simulink model "Fcn1"  (R2017b)
settings: Solver=FixedStepDiscrete  StartTime=0.0  StopTime=10  FixedStep=0.200000  RelTol=1e-3  EnableMultiTasking=on
settings Model: Creator=ktrinh  LastModifiedBy=hbourbou
settings DataIOCC: SaveFormat=Structure
settings OptimizationCC: LifeSpan=inf
settings DebuggingCC: SFUnexpectedBacktrackingDiag=warning  SFNoUnconditionalDefaultTransitionDiag=warning  SFExecutionAtInitializationDiag=none
settings HardwareCC: ProdBitPerSizeT=32  ProdBitPerPtrDiffT=32  ProdWordSize=32  ProdHWDeviceType=Specified
settings CodeAppCC: StateflowObjectComments=on
settings GRTTargetCC: TargetLangStandard=C89/C90 (ANSI)  GeneratePreprocessorConditionals=Disable all
settings ConfigComp: CovMetricSettings=dw  CovHtmlReporting=on  CovSaveCumulativeToWorkspaceVar=on  CovSaveSingleToWorkspaceVar=on  CovExternalEMLEnable=off

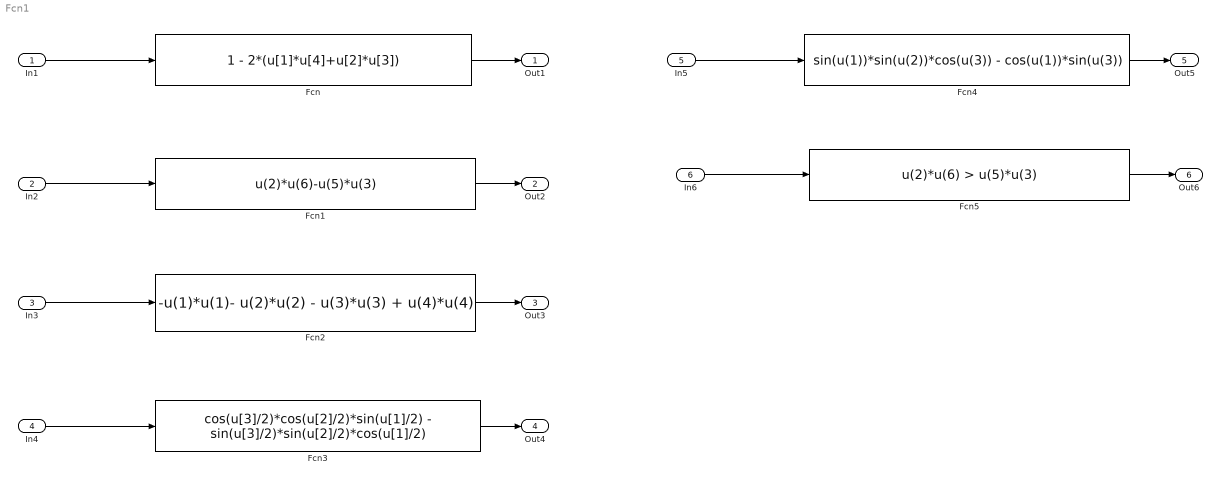
== system Fcn1 ==
  In1 : Inport  PortDimensions=4
  In2 : Inport  Port=2  PortDimensions=6
  In3 : Inport  Port=3  PortDimensions=4
  In4 : Inport  Port=4  PortDimensions=3
  In5 : Inport  Port=5  PortDimensions=3
  In6 : Inport  Port=6  PortDimensions=6
  Fcn : Fcn  Expr=1 - 2*(u[1]*u[4]+u[2]*u[3])
  Fcn1 : Fcn  Expr=u(2)*u(6)-u(5)*u(3)
  Fcn2 : Fcn  Expr=-u(1)*u(1)- u(2)*u(2) - u(3)*u(3) + u(4)*u(4)
  Fcn3 : Fcn  Expr=cos(u[3]/2)*cos(u[2]/2)*sin(u[1]/2) - sin(u[3]/2)*sin(u[2]/2)*cos(u[1]/2)
  Fcn4 : Fcn  Expr=sin(u(1))*sin(u(2))*cos(u(3)) - cos(u(1))*sin(u(3))
  Fcn5 : Fcn  Expr=u(2)*u(6) > u(5)*u(3)
  Out1 : Outport
  Out2 : Outport  Port=2
  Out3 : Outport  Port=3
  Out4 : Outport  Port=4
  Out5 : Outport  Port=5
  Out6 : Outport  Port=6
  wires:
  In1/1 -> Fcn/1
  Fcn/1 -> Out1/1
  Fcn1/1 -> Out2/1
  In2/1 -> Fcn1/1
  In3/1 -> Fcn2/1
  Fcn2/1 -> Out3/1
  Fcn3/1 -> Out4/1
  In4/1 -> Fcn3/1
  Fcn4/1 -> Out5/1
  In5/1 -> Fcn4/1
  In6/1 -> Fcn5/1
  Fcn5/1 -> Out6/1
